simulink model "Impedance_Gantry_Model_V3"  (R2021b)
settings: Solver=VariableStepAuto  StartTime=0  StopTime=5  FixedStep=0.001  RelTol=1e-3  AbsTol=1e-3  EnableMultiTasking=on
values from neighbouring files (symbols this model uses):
  Fmin = obj_x*obj_y*obj_z*obj_density*9.81/obj_coeff/obj_contactpt    (= 4.90500000153)    [Impedance_Control_V1.m]    (also in Impedance_Control_V2.m; Impedance_Control_V3.m; Impedance_Control_V4.m; Impedance_Control_V5.m)
  N = 100    [Gantry_Model_Sim_V1.m]    (also in Impedance_Control_V1.m = 10; Impedance_Control_V2.m = 10; Impedance_Control_V3.m = 40; Impedance_Control_V3_plot.m = 40)
  Ts = 0.01    [Gantry_Model_Sim_V1.m]    (also in Impedance_Control_V1.m = 0.0125; Impedance_Control_V2.m = 0.0125; Impedance_Control_V3.m = 0.0125; Impedance_Control_V4.m = 0.0125)
  z_clear = 1    [Impedance_Control_V1.m]    (also in Impedance_Control_V2.m; Impedance_Control_V3.m; Impedance_Control_V4.m; Impedance_Control_V5.m)
undefined symbols (not defined in the file or in its folder): X, Y, Z
libraries: sm_lib x89, nesl_utility x14, slpidlib x7
(part 3 of 4)

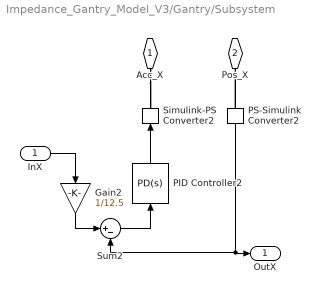
== system Impedance_Gantry_Model_V3/Gantry/Subsystem ==
  InX : Inport
  Gain2 : Gain  Gain=1/12.5
  PID Controller2 : slpidlib/PID Controller  Controller=PD  Form=Parallel  TimeDomain=Continuous-time  UseExternalTs=off  SampleTime=-1  IntegratorMethod=Forward Euler  FilterMethod=Forward Euler  ControllerParametersSource=internal  P=27146.6747627399  I=4557008.73655903  D=1020.02839756073  UseFilter=on  N=1838.86945148368  TunerSelectOption=Transfer Function Based (PID Tuner App)  InitialConditionSource=internal  InitialConditionForIntegrator=0  InitialConditionForFilter=0  DifferentiatorICPrevScaledInput=0  ExternalReset=none  TrackingMode=off  Kt=1  LimitOutput=off  SatLimitsSource=internal  UpperSaturationLimit=inf  LowerSaturationLimit=-inf  LinearizeAsGain=on  AntiWindupMode=none  Kb=1  POutMin=[]  POutMax=[]  IOutMin=[]  IOutMax=[]  DOutMin=[]  DOutMax=[]  NOutMin=[]  NOutMax=[]  SumOutMin=[]  SumOutMax=[]  SaturationOutMin=[]  SaturationOutMax=[]  PParamMin=[]  PParamMax=[]  IParamMin=[]  IParamMax=[]  DParamMin=[]  DParamMax=[]  NParamMin=[]  NParamMax=[]  KbParamMin=[]  KbParamMax=[]  KtParamMin=[]  KtParamMax=[]  KbOutMin=[]  KbOutMax=[]  KtOutMin=[]  KtOutMax=[]  IntegratorOutMin=[]  IntegratorOutMax=[]  FilterOutMin=[]  FilterOutMax=[]  SumI1OutMin=[]  SumI1OutMax=[]  SumI2OutMin=[]  SumI2OutMax=[]  SumI3OutMin=[]  SumI3OutMax=[]  SumI4OutMin=[]  SumI4OutMax=[]  SumDOutMin=[]  SumDOutMax=[]  DifferentiatorOutMin=[]  DifferentiatorOutMax=[]  FilterDiffOutCoefMin=[]  FilterDiffOutCoefMax=[]  ReciprocalOutMin=[]  ReciprocalOutMax=[]  SumDenOutMin=[]  SumDenOutMax=[]  SumNumOutMin=[]  SumNumOutMax=[]  DivideOutMin=[]  DivideOutMax=[]  UdiffTsProdOutMin=[]  UdiffTsProdOutMax=[]  NTsProdOutMin=[]  NTsProdOutMax=[]  UintegralTsProdOutMin=[]  UintegralTsProdOutMax=[]  UngainTsProdOutMin=[]  UngainTsProdOutMax=[]  IntegratorContinuousStateAttributes=''  IntegratorStateMustResolveToSignalObject=off  IntegratorRTWStateStorageClass=Auto  FilterContinuousStateAttributes=''  FilterStateMustResolveToSignalObject=off  FilterRTWStateStorageClass=Auto  ParallelPVariant=InternalParameters  IdealPVariant=Disabled  IVariant=Disabled  DVariant=InternalParameters  IntegratorVariant=Disabled  SatVariant=Disabled  AWVariant=Disabled  PCopyVariant=Disabled  TRVariant=Disabled  FdbkBlocksVariant=Forward  IdealPFdbkVariant=Disabled  SatFdbkVariant=Disabled  DerivativeFilterVariant=ContFilter  NVariant=InternalParameters  NCopyVariant=Disabled  FilterICVariant=InternalICsFilter  IntegratorICVariant=Disabled  ExternalResetVariant=Disabled  TRSumVariant=Passthrough  SumFdbkVariant=Disabled  SumVariant=Sum_PD  TsampFilterVariant=InternalTs  TsampNgainVariant=Passthrough  TsampIntegralVariant=Disabled_SignalSpec  ExternalSaturationOutDataTypeStr=Inherit: Same as second input
  PS-Simulink Converter2 : nesl_utility/PS-Simulink Converter  PhysicalDomain=network_engine_domain  SubClassName=ps_output  LeftPortType=input  RightPortType=output  PseudoPeriodic=off  Frequencies=[]  Unit=inherit  AffineConversion=off
      settings: SourceProductBaseCode=PW,SS
  Simulink-PS Converter2 : nesl_utility/Simulink-PS Converter  PhysicalDomain=network_engine_domain  SubClassName=ps_input  LeftPortType=input  RightPortType=output  PseudoPeriodic=off  Frequencies=[]  NoiseDistribution=none  NoiseParameters=[]  Unit=1  AffineConversion=off  FilteringAndDerivatives=provide  SimscapeFilterOrder=1  InputFilterTimeConstant=0.001  UdotUserProvided=0
      settings: SourceProductBaseCode=PW,SS
  Sum2 : Sum  Inputs=|+-
  Acc_X : PMIOPort  Side=Left
  Pos_X : PMIOPort  Port=2  Side=Right
  OutX : Outport
  wires:
  InX/1 -> Gain2/1
  PS-Simulink Converter2/1 -> OutX/1, Sum2/2
  Sum2/1 -> PID Controller2/1
  PID Controller2/1 -> Simulink-PS Converter2/1
  Gain2/1 -> Sum2/1
  connections:
  PS-Simulink Converter2/LConn1 -- Pos_X/RConn1
  Acc_X/RConn1 -- Simulink-PS Converter2/RConn1

== system Impedance_Gantry_Model_V3/Gantry/Y axis dynamics ==
  InY : Inport
  Gain1 : Gain  Gain=1/500
  PID Controller1 : slpidlib/PID Controller  Controller=PD  Form=Parallel  TimeDomain=Continuous-time  UseExternalTs=off  SampleTime=-1  IntegratorMethod=Forward Euler  FilterMethod=Forward Euler  ControllerParametersSource=internal  P=131139.225952649  I=4557008.73655903  D=1480.57986826149  UseFilter=on  N=47126.9268470762  TunerSelectOption=Transfer Function Based (PID Tuner App)  InitialConditionSource=internal  InitialConditionForIntegrator=0  InitialConditionForFilter=0  DifferentiatorICPrevScaledInput=0  ExternalReset=none  TrackingMode=off  Kt=1  LimitOutput=off  SatLimitsSource=internal  UpperSaturationLimit=inf  LowerSaturationLimit=-inf  LinearizeAsGain=on  AntiWindupMode=none  Kb=1  POutMin=[]  POutMax=[]  IOutMin=[]  IOutMax=[]  DOutMin=[]  DOutMax=[]  NOutMin=[]  NOutMax=[]  SumOutMin=[]  SumOutMax=[]  SaturationOutMin=[]  SaturationOutMax=[]  PParamMin=[]  PParamMax=[]  IParamMin=[]  IParamMax=[]  DParamMin=[]  DParamMax=[]  NParamMin=[]  NParamMax=[]  KbParamMin=[]  KbParamMax=[]  KtParamMin=[]  KtParamMax=[]  KbOutMin=[]  KbOutMax=[]  KtOutMin=[]  KtOutMax=[]  IntegratorOutMin=[]  IntegratorOutMax=[]  FilterOutMin=[]  FilterOutMax=[]  SumI1OutMin=[]  SumI1OutMax=[]  SumI2OutMin=[]  SumI2OutMax=[]  SumI3OutMin=[]  SumI3OutMax=[]  SumI4OutMin=[]  SumI4OutMax=[]  SumDOutMin=[]  SumDOutMax=[]  DifferentiatorOutMin=[]  DifferentiatorOutMax=[]  FilterDiffOutCoefMin=[]  FilterDiffOutCoefMax=[]  ReciprocalOutMin=[]  ReciprocalOutMax=[]  SumDenOutMin=[]  SumDenOutMax=[]  SumNumOutMin=[]  SumNumOutMax=[]  DivideOutMin=[]  DivideOutMax=[]  UdiffTsProdOutMin=[]  UdiffTsProdOutMax=[]  NTsProdOutMin=[]  NTsProdOutMax=[]  UintegralTsProdOutMin=[]  UintegralTsProdOutMax=[]  UngainTsProdOutMin=[]  UngainTsProdOutMax=[]  IntegratorContinuousStateAttributes=''  IntegratorStateMustResolveToSignalObject=off  IntegratorRTWStateStorageClass=Auto  FilterContinuousStateAttributes=''  FilterStateMustResolveToSignalObject=off  FilterRTWStateStorageClass=Auto  ParallelPVariant=InternalParameters  IdealPVariant=Disabled  IVariant=Disabled  DVariant=InternalParameters  IntegratorVariant=Disabled  SatVariant=Disabled  AWVariant=Disabled  PCopyVariant=Disabled  TRVariant=Disabled  FdbkBlocksVariant=Forward  IdealPFdbkVariant=Disabled  SatFdbkVariant=Disabled  DerivativeFilterVariant=ContFilter  NVariant=InternalParameters  NCopyVariant=Disabled  FilterICVariant=InternalICsFilter  IntegratorICVariant=Disabled  ExternalResetVariant=Disabled  TRSumVariant=Passthrough  SumFdbkVariant=Disabled  SumVariant=Sum_PD  TsampFilterVariant=InternalTs  TsampNgainVariant=Passthrough  TsampIntegralVariant=Disabled_SignalSpec  ExternalSaturationOutDataTypeStr=Inherit: Same as second input
  PS-Simulink Converter1 : nesl_utility/PS-Simulink Converter  PhysicalDomain=network_engine_domain  SubClassName=ps_output  LeftPortType=input  RightPortType=output  PseudoPeriodic=off  Frequencies=[]  Unit=inherit  AffineConversion=off
      settings: SourceProductBaseCode=PW,SS
  Simulink-PS Converter1 : nesl_utility/Simulink-PS Converter  PhysicalDomain=network_engine_domain  SubClassName=ps_input  LeftPortType=input  RightPortType=output  PseudoPeriodic=off  Frequencies=[]  NoiseDistribution=none  NoiseParameters=[]  Unit=1  AffineConversion=off  FilteringAndDerivatives=provide  SimscapeFilterOrder=1  InputFilterTimeConstant=0.001  UdotUserProvided=0
      settings: SourceProductBaseCode=PW,SS
  Sum1 : Sum  Inputs=|+-
  Acc_Y : PMIOPort  Side=Left
  Pos_Y : PMIOPort  Port=2  Side=Right
  OutY : Outport
  wires:
  Gain1/1 -> Sum1/1
  PID Controller1/1 -> Simulink-PS Converter1/1
  PS-Simulink Converter1/1 -> Sum1/2, OutY/1
  InY/1 -> Gain1/1
  Sum1/1 -> PID Controller1/1
  connections:
  Pos_Y/RConn1 -- PS-Simulink Converter1/LConn1
  Simulink-PS Converter1/RConn1 -- Acc_Y/RConn1

== system Impedance_Gantry_Model_V3/Gantry/Z axis dynamics ==
  InZ : Inport
  Gain : Gain  Gain=1/1550.672269
  PID Controller : slpidlib/PID Controller  Controller=PD  Form=Parallel  TimeDomain=Continuous-time  UseExternalTs=off  SampleTime=-1  IntegratorMethod=Forward Euler  FilterMethod=Forward Euler  ControllerParametersSource=internal  P=33734.3806  I=809967.572319892  D=163.3421  UseFilter=on  N=13723.0524  TunerSelectOption=Transfer Function Based (PID Tuner App)  InitialConditionSource=internal  InitialConditionForIntegrator=0  InitialConditionForFilter=0  DifferentiatorICPrevScaledInput=0  ExternalReset=none  TrackingMode=off  Kt=1  LimitOutput=off  SatLimitsSource=internal  UpperSaturationLimit=inf  LowerSaturationLimit=-inf  LinearizeAsGain=on  AntiWindupMode=none  Kb=1  POutMin=[]  POutMax=[]  IOutMin=[]  IOutMax=[]  DOutMin=[]  DOutMax=[]  NOutMin=[]  NOutMax=[]  SumOutMin=[]  SumOutMax=[]  SaturationOutMin=[]  SaturationOutMax=[]  PParamMin=[]  PParamMax=[]  IParamMin=[]  IParamMax=[]  DParamMin=[]  DParamMax=[]  NParamMin=[]  NParamMax=[]  KbParamMin=[]  KbParamMax=[]  KtParamMin=[]  KtParamMax=[]  KbOutMin=[]  KbOutMax=[]  KtOutMin=[]  KtOutMax=[]  IntegratorOutMin=[]  IntegratorOutMax=[]  FilterOutMin=[]  FilterOutMax=[]  SumI1OutMin=[]  SumI1OutMax=[]  SumI2OutMin=[]  SumI2OutMax=[]  SumI3OutMin=[]  SumI3OutMax=[]  SumI4OutMin=[]  SumI4OutMax=[]  SumDOutMin=[]  SumDOutMax=[]  DifferentiatorOutMin=[]  DifferentiatorOutMax=[]  FilterDiffOutCoefMin=[]  FilterDiffOutCoefMax=[]  ReciprocalOutMin=[]  ReciprocalOutMax=[]  SumDenOutMin=[]  SumDenOutMax=[]  SumNumOutMin=[]  SumNumOutMax=[]  DivideOutMin=[]  DivideOutMax=[]  UdiffTsProdOutMin=[]  UdiffTsProdOutMax=[]  NTsProdOutMin=[]  NTsProdOutMax=[]  UintegralTsProdOutMin=[]  UintegralTsProdOutMax=[]  UngainTsProdOutMin=[]  UngainTsProdOutMax=[]  IntegratorContinuousStateAttributes=''  IntegratorStateMustResolveToSignalObject=off  IntegratorRTWStateStorageClass=Auto  FilterContinuousStateAttributes=''  FilterStateMustResolveToSignalObject=off  FilterRTWStateStorageClass=Auto  ParallelPVariant=InternalParameters  IdealPVariant=Disabled  IVariant=Disabled  DVariant=InternalParameters  IntegratorVariant=Disabled  SatVariant=Disabled  AWVariant=Disabled  PCopyVariant=Disabled  TRVariant=Disabled  FdbkBlocksVariant=Forward  IdealPFdbkVariant=Disabled  SatFdbkVariant=Disabled  DerivativeFilterVariant=ContFilter  NVariant=InternalParameters  NCopyVariant=Disabled  FilterICVariant=InternalICsFilter  IntegratorICVariant=Disabled  ExternalResetVariant=Disabled  TRSumVariant=Passthrough  SumFdbkVariant=Disabled  SumVariant=Sum_PD  TsampFilterVariant=InternalTs  TsampNgainVariant=Passthrough  TsampIntegralVariant=Disabled_SignalSpec  ExternalSaturationOutDataTypeStr=Inherit: Same as second input
  PS-Simulink Converter : nesl_utility/PS-Simulink Converter  PhysicalDomain=network_engine_domain  SubClassName=ps_output  LeftPortType=input  RightPortType=output  PseudoPeriodic=off  Frequencies=[]  Unit=inherit  AffineConversion=off
      settings: SourceProductBaseCode=PW,SS
  Simulink-PS Converter : nesl_utility/Simulink-PS Converter  PhysicalDomain=network_engine_domain  SubClassName=ps_input  LeftPortType=input  RightPortType=output  PseudoPeriodic=off  Frequencies=[]  NoiseDistribution=none  NoiseParameters=[]  Unit=1  AffineConversion=off  FilteringAndDerivatives=provide  SimscapeFilterOrder=1  InputFilterTimeConstant=0.001  UdotUserProvided=0
      settings: SourceProductBaseCode=PW,SS
  Sum : Sum  Inputs=|+-
  Acc_Z : PMIOPort  Side=Left
  Pos_Z : PMIOPort  Port=2  Side=Right
  OutZ : Outport
  wires:
  Sum/1 -> PID Controller/1
  PS-Simulink Converter/1 -> OutZ/1, Sum/2
  PID Controller/1 -> Simulink-PS Converter/1
  Gain/1 -> Sum/1
  InZ/1 -> Gain/1
  connections:
  PS-Simulink Converter/LConn1 -- Pos_Z/RConn1
  Simulink-PS Converter/RConn1 -- Acc_Z/RConn1

== system Impedance_Gantry_Model_V3/Gantry/Z axis dynamics1 ==
  InZ : Inport
  Gain : Gain  Gain=1/1550.672269
  PID Controller : slpidlib/PID Controller  Controller=PD  Form=Parallel  TimeDomain=Continuous-time  UseExternalTs=off  SampleTime=-1  IntegratorMethod=Forward Euler  FilterMethod=Forward Euler  ControllerParametersSource=internal  P=33734.3806  I=809967.572319892  D=163.3421  UseFilter=on  N=13723.0524  TunerSelectOption=Transfer Function Based (PID Tuner App)  InitialConditionSource=internal  InitialConditionForIntegrator=0  InitialConditionForFilter=0  DifferentiatorICPrevScaledInput=0  ExternalReset=none  TrackingMode=off  Kt=1  LimitOutput=off  SatLimitsSource=internal  UpperSaturationLimit=inf  LowerSaturationLimit=-inf  LinearizeAsGain=on  AntiWindupMode=none  Kb=1  POutMin=[]  POutMax=[]  IOutMin=[]  IOutMax=[]  DOutMin=[]  DOutMax=[]  NOutMin=[]  NOutMax=[]  SumOutMin=[]  SumOutMax=[]  SaturationOutMin=[]  SaturationOutMax=[]  PParamMin=[]  PParamMax=[]  IParamMin=[]  IParamMax=[]  DParamMin=[]  DParamMax=[]  NParamMin=[]  NParamMax=[]  KbParamMin=[]  KbParamMax=[]  KtParamMin=[]  KtParamMax=[]  KbOutMin=[]  KbOutMax=[]  KtOutMin=[]  KtOutMax=[]  IntegratorOutMin=[]  IntegratorOutMax=[]  FilterOutMin=[]  FilterOutMax=[]  SumI1OutMin=[]  SumI1OutMax=[]  SumI2OutMin=[]  SumI2OutMax=[]  SumI3OutMin=[]  SumI3OutMax=[]  SumI4OutMin=[]  SumI4OutMax=[]  SumDOutMin=[]  SumDOutMax=[]  DifferentiatorOutMin=[]  DifferentiatorOutMax=[]  FilterDiffOutCoefMin=[]  FilterDiffOutCoefMax=[]  ReciprocalOutMin=[]  ReciprocalOutMax=[]  SumDenOutMin=[]  SumDenOutMax=[]  SumNumOutMin=[]  SumNumOutMax=[]  DivideOutMin=[]  DivideOutMax=[]  UdiffTsProdOutMin=[]  UdiffTsProdOutMax=[]  NTsProdOutMin=[]  NTsProdOutMax=[]  UintegralTsProdOutMin=[]  UintegralTsProdOutMax=[]  UngainTsProdOutMin=[]  UngainTsProdOutMax=[]  IntegratorContinuousStateAttributes=''  IntegratorStateMustResolveToSignalObject=off  IntegratorRTWStateStorageClass=Auto  FilterContinuousStateAttributes=''  FilterStateMustResolveToSignalObject=off  FilterRTWStateStorageClass=Auto  ParallelPVariant=InternalParameters  IdealPVariant=Disabled  IVariant=Disabled  DVariant=InternalParameters  IntegratorVariant=Disabled  SatVariant=Disabled  AWVariant=Disabled  PCopyVariant=Disabled  TRVariant=Disabled  FdbkBlocksVariant=Forward  IdealPFdbkVariant=Disabled  SatFdbkVariant=Disabled  DerivativeFilterVariant=ContFilter  NVariant=InternalParameters  NCopyVariant=Disabled  FilterICVariant=InternalICsFilter  IntegratorICVariant=Disabled  ExternalResetVariant=Disabled  TRSumVariant=Passthrough  SumFdbkVariant=Disabled  SumVariant=Sum_PD  TsampFilterVariant=InternalTs  TsampNgainVariant=Passthrough  TsampIntegralVariant=Disabled_SignalSpec  ExternalSaturationOutDataTypeStr=Inherit: Same as second input
  PS-Simulink Converter : nesl_utility/PS-Simulink Converter  PhysicalDomain=network_engine_domain  SubClassName=ps_output  LeftPortType=input  RightPortType=output  PseudoPeriodic=off  Frequencies=[]  Unit=inherit  AffineConversion=off
      settings: SourceProductBaseCode=PW,SS
  Simulink-PS Converter : nesl_utility/Simulink-PS Converter  PhysicalDomain=network_engine_domain  SubClassName=ps_input  LeftPortType=input  RightPortType=output  PseudoPeriodic=off  Frequencies=[]  NoiseDistribution=none  NoiseParameters=[]  Unit=1  AffineConversion=off  FilteringAndDerivatives=provide  SimscapeFilterOrder=1  InputFilterTimeConstant=0.001  UdotUserProvided=0
      settings: SourceProductBaseCode=PW,SS
  Sum : Sum  Inputs=|+-
  Acc_Z : PMIOPort  Side=Left
  Pos_Z : PMIOPort  Port=2  Side=Right
  OutZ : Outport
  wires:
  Sum/1 -> PID Controller/1
  PS-Simulink Converter/1 -> OutZ/1, Sum/2
  PID Controller/1 -> Simulink-PS Converter/1
  Gain/1 -> Sum/1
  InZ/1 -> Gain/1
  connections:
  PS-Simulink Converter/LConn1 -- Pos_Z/RConn1
  Simulink-PS Converter/RConn1 -- Acc_Z/RConn1

== system Impedance_Gantry_Model_V3/Gantry/Z axis dynamics2 ==
  InZ : Inport
  Gain : Gain  Gain=1/1550.672269
  PID Controller : slpidlib/PID Controller  Controller=PD  Form=Parallel  TimeDomain=Continuous-time  UseExternalTs=off  SampleTime=-1  IntegratorMethod=Forward Euler  FilterMethod=Forward Euler  ControllerParametersSource=internal  P=33734.3806  I=809967.572319892  D=163.3421  UseFilter=on  N=13723.0524  TunerSelectOption=Transfer Function Based (PID Tuner App)  InitialConditionSource=internal  InitialConditionForIntegrator=0  InitialConditionForFilter=0  DifferentiatorICPrevScaledInput=0  ExternalReset=none  TrackingMode=off  Kt=1  LimitOutput=off  SatLimitsSource=internal  UpperSaturationLimit=inf  LowerSaturationLimit=-inf  LinearizeAsGain=on  AntiWindupMode=none  Kb=1  POutMin=[]  POutMax=[]  IOutMin=[]  IOutMax=[]  DOutMin=[]  DOutMax=[]  NOutMin=[]  NOutMax=[]  SumOutMin=[]  SumOutMax=[]  SaturationOutMin=[]  SaturationOutMax=[]  PParamMin=[]  PParamMax=[]  IParamMin=[]  IParamMax=[]  DParamMin=[]  DParamMax=[]  NParamMin=[]  NParamMax=[]  KbParamMin=[]  KbParamMax=[]  KtParamMin=[]  KtParamMax=[]  KbOutMin=[]  KbOutMax=[]  KtOutMin=[]  KtOutMax=[]  IntegratorOutMin=[]  IntegratorOutMax=[]  FilterOutMin=[]  FilterOutMax=[]  SumI1OutMin=[]  SumI1OutMax=[]  SumI2OutMin=[]  SumI2OutMax=[]  SumI3OutMin=[]  SumI3OutMax=[]  SumI4OutMin=[]  SumI4OutMax=[]  SumDOutMin=[]  SumDOutMax=[]  DifferentiatorOutMin=[]  DifferentiatorOutMax=[]  FilterDiffOutCoefMin=[]  FilterDiffOutCoefMax=[]  ReciprocalOutMin=[]  ReciprocalOutMax=[]  SumDenOutMin=[]  SumDenOutMax=[]  SumNumOutMin=[]  SumNumOutMax=[]  DivideOutMin=[]  DivideOutMax=[]  UdiffTsProdOutMin=[]  UdiffTsProdOutMax=[]  NTsProdOutMin=[]  NTsProdOutMax=[]  UintegralTsProdOutMin=[]  UintegralTsProdOutMax=[]  UngainTsProdOutMin=[]  UngainTsProdOutMax=[]  IntegratorContinuousStateAttributes=''  IntegratorStateMustResolveToSignalObject=off  IntegratorRTWStateStorageClass=Auto  FilterContinuousStateAttributes=''  FilterStateMustResolveToSignalObject=off  FilterRTWStateStorageClass=Auto  ParallelPVariant=InternalParameters  IdealPVariant=Disabled  IVariant=Disabled  DVariant=InternalParameters  IntegratorVariant=Disabled  SatVariant=Disabled  AWVariant=Disabled  PCopyVariant=Disabled  TRVariant=Disabled  FdbkBlocksVariant=Forward  IdealPFdbkVariant=Disabled  SatFdbkVariant=Disabled  DerivativeFilterVariant=ContFilter  NVariant=InternalParameters  NCopyVariant=Disabled  FilterICVariant=InternalICsFilter  IntegratorICVariant=Disabled  ExternalResetVariant=Disabled  TRSumVariant=Passthrough  SumFdbkVariant=Disabled  SumVariant=Sum_PD  TsampFilterVariant=InternalTs  TsampNgainVariant=Passthrough  TsampIntegralVariant=Disabled_SignalSpec  ExternalSaturationOutDataTypeStr=Inherit: Same as second input
  PS-Simulink Converter : nesl_utility/PS-Simulink Converter  PhysicalDomain=network_engine_domain  SubClassName=ps_output  LeftPortType=input  RightPortType=output  PseudoPeriodic=off  Frequencies=[]  Unit=inherit  AffineConversion=off
      settings: SourceProductBaseCode=PW,SS
  Simulink-PS Converter : nesl_utility/Simulink-PS Converter  PhysicalDomain=network_engine_domain  SubClassName=ps_input  LeftPortType=input  RightPortType=output  PseudoPeriodic=off  Frequencies=[]  NoiseDistribution=none  NoiseParameters=[]  Unit=1  AffineConversion=off  FilteringAndDerivatives=provide  SimscapeFilterOrder=1  InputFilterTimeConstant=0.001  UdotUserProvided=0
      settings: SourceProductBaseCode=PW,SS
  Sum : Sum  Inputs=|+-
  Acc_Z : PMIOPort  Side=Left
  Pos_Z : PMIOPort  Port=2  Side=Right
  OutZ : Outport
  wires:
  Sum/1 -> PID Controller/1
  PS-Simulink Converter/1 -> OutZ/1, Sum/2
  PID Controller/1 -> Simulink-PS Converter/1
  Gain/1 -> Sum/1
  InZ/1 -> Gain/1
  connections:
  PS-Simulink Converter/LConn1 -- Pos_Z/RConn1
  Simulink-PS Converter/RConn1 -- Acc_Z/RConn1

== system Impedance_Gantry_Model_V3/ObjectAndEnviroment/BBL ==
  BBL : sm_lib/Frames and Transforms/Rigid Transform  TranslationMethod=Cartesian  TranslationStandardOffset=0  TranslationLengthUnit=mm  TranslationStandardAxis=+Z  TranslationCartesianOffset=[25 25 0]  TranslationROffset=0  TranslationROffsetUnits=m  TranslationZOffset=0  TranslationZOffsetUnits=m  TranslationThetaOffset=0  TranslationThetaOffsetUnits=deg  RotationMethod=None  RotationAngleUnits=deg  RotationStandardAxis=+Z  RotationAngle=0.0  RotationArbitraryAxis=[0 0 1]  FollAlignAxisA=+X  BaseAlignAxisA=+Y  FollAlignAxisB=+Y  BaseAlignAxisB=+Z  RotationSequenceAxes=FollowerAxes  RotationSequence=XYX  RotationSequenceAngles=[0 0 0]  RotationSequenceAnglesUnits=deg  RotationMatrix=[1 0 0; 0 1 0; 0 0 1]
  BBLBall : sm_lib/Body Elements/Spherical Solid  GraphicAmbientColor=[0.15 0.15 0.15 1.0]  BasedOnType=Density  CenterOfMass=[0 0 0]  CenterOfMassUnits=m  GraphicDiffuseColor=[0.5 0.5 0.5]  Density=1000  DensityUnits=kg/m^3  DoExposeReferenceFrame=on  GraphicEmissiveColor=[0.0 0.0 0.0 1.0]  ExportEntireGeometry=on  SerializedExposedGeometries=<ExposedGeometries><ExposedGeometry><RawGeometryId>entire</RawGeometryId><ExposedGeometryId>G</ExposedGeometryId></ExposedGeometry></ExposedGeometries>  SerializedFrames=<Frames/>  MarkerShape=Sphere  MarkerSize=10  GraphicType=FromGeometry  InertiaType=CalculateFromGeometry  Mass=1  MassUnits=kg  MomentsOfInertia=[1 1 1]  MomentsOfInertiaUnits=kg*m^2  GraphicOpacity=1.0  ProductsOfInertia=[0 0 0]  ProductsOfInertiaUnits=kg*m^2  GraphicShininess=75  GraphicSpecularColor=[0.5 0.5 0.5 1.0]  SphereRadius=1  SphereRadiusUnits=mm  GraphicVisPropType=SimpleVisualProperties
  BBLConveyerDest : sm_lib/Forces and Torques/Spatial Contact Force  CoefficientOfDynamicFriction=0.5  CoefficientOfStaticFriction=0.5  SenseContactBaseRotation=off  SenseContactBaseTranslation=off  NormalDamping=30  NormalDampingUnits=N/(m/s)  SenseContactFollowerRotation=off  SenseContactFollowerTranslation=off  SenseContactSignal=off  NormalStiffness=1e4  NormalStiffnessUnits=N/m  FrictionalCriticalVelocity=1e-3  FrictionalCriticalVelocityUnits=m/s  ZeroCrossDetectContactStartAndEnd=off  FrictionType=SmoothStickSlip  SenseFrictionalForceMagnitude=off  SenseNormalForceMagnitude=off  NormalForceType=SmoothSpringDamper  SenseNormalVelocity=off  SenseSeparationDistance=off  SenseTangentialVelocity=off  SenseTangentialVelocityMagnitude=off  NormalTransitionRegionWidth=1e-5  NormalTransitionRegionWidthUnits=m
  BBLConveyerOri : sm_lib/Forces and Torques/Spatial Contact Force  CoefficientOfDynamicFriction=0.5  CoefficientOfStaticFriction=0.5  SenseContactBaseRotation=off  SenseContactBaseTranslation=off  NormalDamping=30  NormalDampingUnits=N/(m/s)  SenseContactFollowerRotation=off  SenseContactFollowerTranslation=off  SenseContactSignal=off  NormalStiffness=1e4  NormalStiffnessUnits=N/m  FrictionalCriticalVelocity=1e-3  FrictionalCriticalVelocityUnits=m/s  ZeroCrossDetectContactStartAndEnd=off  FrictionType=SmoothStickSlip  SenseFrictionalForceMagnitude=off  SenseNormalForceMagnitude=off  NormalForceType=SmoothSpringDamper  SenseNormalVelocity=off  SenseSeparationDistance=off  SenseTangentialVelocity=off  SenseTangentialVelocityMagnitude=off  NormalTransitionRegionWidth=1e-5  NormalTransitionRegionWidthUnits=m
  BBLGripper : sm_lib/Forces and Torques/Spatial Contact Force  CoefficientOfDynamicFriction=0.5  CoefficientOfStaticFriction=0.5  SenseContactBaseRotation=off  SenseContactBaseTranslation=off  NormalDamping=0  NormalDampingUnits=N/(m/s)  SenseContactFollowerRotation=off  SenseContactFollowerTranslation=off  SenseContactSignal=off  NormalStiffness=1e4  NormalStiffnessUnits=N/m  FrictionalCriticalVelocity=1e-3  FrictionalCriticalVelocityUnits=m/s  ZeroCrossDetectContactStartAndEnd=off  FrictionType=SmoothStickSlip  SenseFrictionalForceMagnitude=off  SenseNormalForceMagnitude=off  NormalForceType=SmoothSpringDamper  SenseNormalVelocity=off  SenseSeparationDistance=off  SenseTangentialVelocity=off  SenseTangentialVelocityMagnitude=off  NormalTransitionRegionWidth=1e-5  NormalTransitionRegionWidthUnits=m
  Obj : PMIOPort  Side=Left
  Gripper : PMIOPort  Port=2  Side=Right
  ConveyerOri : PMIOPort  Port=3  Side=Right
  ConveyerDest : PMIOPort  Port=4  Side=Right
  connections:
  BBLBall/LConn1 -- BBLConveyerDest/LConn1 -- BBLConveyerOri/LConn1 -- BBLGripper/LConn1
  BBL/LConn1 -- Obj/RConn1
  BBLBall/RConn1 -- BBL/RConn1
  ConveyerOri/RConn1 -- BBLConveyerOri/RConn1
  BBLGripper/RConn1 -- Gripper/RConn1
  BBLConveyerDest/RConn1 -- ConveyerDest/RConn1

== system Impedance_Gantry_Model_V3/ObjectAndEnviroment/BRR ==
  BBR : sm_lib/Frames and Transforms/Rigid Transform  TranslationMethod=Cartesian  TranslationStandardOffset=0  TranslationLengthUnit=mm  TranslationStandardAxis=+Z  TranslationCartesianOffset=[25 0 0]  TranslationROffset=0  TranslationROffsetUnits=m  TranslationZOffset=0  TranslationZOffsetUnits=m  TranslationThetaOffset=0  TranslationThetaOffsetUnits=deg  RotationMethod=None  RotationAngleUnits=deg  RotationStandardAxis=+Z  RotationAngle=0.0  RotationArbitraryAxis=[0 0 1]  FollAlignAxisA=+X  BaseAlignAxisA=+Y  FollAlignAxisB=+Y  BaseAlignAxisB=+Z  RotationSequenceAxes=FollowerAxes  RotationSequence=XYX  RotationSequenceAngles=[0 0 0]  RotationSequenceAnglesUnits=deg  RotationMatrix=[1 0 0; 0 1 0; 0 0 1]
  BBRBall : sm_lib/Body Elements/Spherical Solid  GraphicAmbientColor=[0.15 0.15 0.15 1.0]  BasedOnType=Density  CenterOfMass=[0 0 0]  CenterOfMassUnits=m  GraphicDiffuseColor=[0.5 0.5 0.5]  Density=1000  DensityUnits=kg/m^3  DoExposeReferenceFrame=on  GraphicEmissiveColor=[0.0 0.0 0.0 1.0]  ExportEntireGeometry=on  SerializedExposedGeometries=<ExposedGeometries><ExposedGeometry><RawGeometryId>entire</RawGeometryId><ExposedGeometryId>G</ExposedGeometryId></ExposedGeometry></ExposedGeometries>  SerializedFrames=<Frames/>  MarkerShape=Sphere  MarkerSize=10  GraphicType=FromGeometry  InertiaType=CalculateFromGeometry  Mass=1  MassUnits=kg  MomentsOfInertia=[1 1 1]  MomentsOfInertiaUnits=kg*m^2  GraphicOpacity=1.0  ProductsOfInertia=[0 0 0]  ProductsOfInertiaUnits=kg*m^2  GraphicShininess=75  GraphicSpecularColor=[0.5 0.5 0.5 1.0]  SphereRadius=1  SphereRadiusUnits=mm  GraphicVisPropType=SimpleVisualProperties
  BBRConveyerDest : sm_lib/Forces and Torques/Spatial Contact Force  CoefficientOfDynamicFriction=0.5  CoefficientOfStaticFriction=0.5  SenseContactBaseRotation=off  SenseContactBaseTranslation=off  NormalDamping=30  NormalDampingUnits=N/(m/s)  SenseContactFollowerRotation=off  SenseContactFollowerTranslation=off  SenseContactSignal=off  NormalStiffness=1e4  NormalStiffnessUnits=N/m  FrictionalCriticalVelocity=1e-3  FrictionalCriticalVelocityUnits=m/s  ZeroCrossDetectContactStartAndEnd=off  FrictionType=SmoothStickSlip  SenseFrictionalForceMagnitude=off  SenseNormalForceMagnitude=off  NormalForceType=SmoothSpringDamper  SenseNormalVelocity=off  SenseSeparationDistance=off  SenseTangentialVelocity=off  SenseTangentialVelocityMagnitude=off  NormalTransitionRegionWidth=1e-5  NormalTransitionRegionWidthUnits=m
  BBRConveyerOri : sm_lib/Forces and Torques/Spatial Contact Force  CoefficientOfDynamicFriction=0.5  CoefficientOfStaticFriction=0.5  SenseContactBaseRotation=off  SenseContactBaseTranslation=off  NormalDamping=30  NormalDampingUnits=N/(m/s)  SenseContactFollowerRotation=off  SenseContactFollowerTranslation=off  SenseContactSignal=off  NormalStiffness=1e4  NormalStiffnessUnits=N/m  FrictionalCriticalVelocity=1e-3  FrictionalCriticalVelocityUnits=m/s  ZeroCrossDetectContactStartAndEnd=off  FrictionType=SmoothStickSlip  SenseFrictionalForceMagnitude=off  SenseNormalForceMagnitude=off  NormalForceType=SmoothSpringDamper  SenseNormalVelocity=off  SenseSeparationDistance=off  SenseTangentialVelocity=off  SenseTangentialVelocityMagnitude=off  NormalTransitionRegionWidth=1e-5  NormalTransitionRegionWidthUnits=m
  BBRGripper : sm_lib/Forces and Torques/Spatial Contact Force  CoefficientOfDynamicFriction=0.5  CoefficientOfStaticFriction=0.5  SenseContactBaseRotation=off  SenseContactBaseTranslation=off  NormalDamping=0  NormalDampingUnits=N/(m/s)  SenseContactFollowerRotation=off  SenseContactFollowerTranslation=off  SenseContactSignal=off  NormalStiffness=1e4  NormalStiffnessUnits=N/m  FrictionalCriticalVelocity=1e-3  FrictionalCriticalVelocityUnits=m/s  ZeroCrossDetectContactStartAndEnd=off  FrictionType=SmoothStickSlip  SenseFrictionalForceMagnitude=off  SenseNormalForceMagnitude=off  NormalForceType=SmoothSpringDamper  SenseNormalVelocity=off  SenseSeparationDistance=off  SenseTangentialVelocity=off  SenseTangentialVelocityMagnitude=off  NormalTransitionRegionWidth=1e-5  NormalTransitionRegionWidthUnits=m
  Obj : PMIOPort  Side=Left
  Gripper : PMIOPort  Port=2  Side=Right
  ConveyerOri : PMIOPort  Port=3  Side=Right
  ConveyerDest : PMIOPort  Port=4  Side=Right
  connections:
  BBRBall/LConn1 -- BBRConveyerDest/LConn1 -- BBRConveyerOri/LConn1 -- BBRGripper/LConn1
  ConveyerOri/RConn1 -- BBRConveyerOri/RConn1
  BBRBall/RConn1 -- BBR/RConn1
  Gripper/RConn1 -- BBRGripper/RConn1
  BBR/LConn1 -- Obj/RConn1
  BBRConveyerDest/RConn1 -- ConveyerDest/RConn1

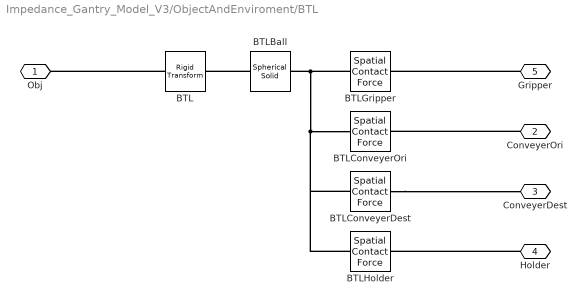
== system Impedance_Gantry_Model_V3/ObjectAndEnviroment/BTL ==
  BTL : sm_lib/Frames and Transforms/Rigid Transform  TranslationMethod=Cartesian  TranslationStandardOffset=0  TranslationLengthUnit=mm  TranslationStandardAxis=+Z  TranslationCartesianOffset=[25 25 30]  TranslationROffset=0  TranslationROffsetUnits=m  TranslationZOffset=0  TranslationZOffsetUnits=m  TranslationThetaOffset=0  TranslationThetaOffsetUnits=deg  RotationMethod=None  RotationAngleUnits=deg  RotationStandardAxis=+Z  RotationAngle=0.0  RotationArbitraryAxis=[0 0 1]  FollAlignAxisA=+X  BaseAlignAxisA=+Y  FollAlignAxisB=+Y  BaseAlignAxisB=+Z  RotationSequenceAxes=FollowerAxes  RotationSequence=XYX  RotationSequenceAngles=[0 0 0]  RotationSequenceAnglesUnits=deg  RotationMatrix=[1 0 0; 0 1 0; 0 0 1]
  BTLBall : sm_lib/Body Elements/Spherical Solid  GraphicAmbientColor=[0.15 0.15 0.15 1.0]  BasedOnType=Density  CenterOfMass=[0 0 0]  CenterOfMassUnits=m  GraphicDiffuseColor=[0.5 0.5 0.5]  Density=1000  DensityUnits=kg/m^3  DoExposeReferenceFrame=on  GraphicEmissiveColor=[0.0 0.0 0.0 1.0]  ExportEntireGeometry=on  SerializedExposedGeometries=<ExposedGeometries><ExposedGeometry><RawGeometryId>entire</RawGeometryId><ExposedGeometryId>G</ExposedGeometryId></ExposedGeometry></ExposedGeometries>  SerializedFrames=<Frames/>  MarkerShape=Sphere  MarkerSize=10  GraphicType=FromGeometry  InertiaType=CalculateFromGeometry  Mass=1  MassUnits=kg  MomentsOfInertia=[1 1 1]  MomentsOfInertiaUnits=kg*m^2  GraphicOpacity=1.0  ProductsOfInertia=[0 0 0]  ProductsOfInertiaUnits=kg*m^2  GraphicShininess=75  GraphicSpecularColor=[0.5 0.5 0.5 1.0]  SphereRadius=1  SphereRadiusUnits=mm  GraphicVisPropType=SimpleVisualProperties
  BTLConveyerDest : sm_lib/Forces and Torques/Spatial Contact Force  CoefficientOfDynamicFriction=0.5  CoefficientOfStaticFriction=0.5  SenseContactBaseRotation=off  SenseContactBaseTranslation=off  NormalDamping=30  NormalDampingUnits=N/(m/s)  SenseContactFollowerRotation=off  SenseContactFollowerTranslation=off  SenseContactSignal=off  NormalStiffness=1e4  NormalStiffnessUnits=N/m  FrictionalCriticalVelocity=1e-3  FrictionalCriticalVelocityUnits=m/s  ZeroCrossDetectContactStartAndEnd=off  FrictionType=SmoothStickSlip  SenseFrictionalForceMagnitude=off  SenseNormalForceMagnitude=off  NormalForceType=SmoothSpringDamper  SenseNormalVelocity=off  SenseSeparationDistance=off  SenseTangentialVelocity=off  SenseTangentialVelocityMagnitude=off  NormalTransitionRegionWidth=1e-5  NormalTransitionRegionWidthUnits=m
  BTLConveyerOri : sm_lib/Forces and Torques/Spatial Contact Force  CoefficientOfDynamicFriction=0.5  CoefficientOfStaticFriction=0.5  SenseContactBaseRotation=off  SenseContactBaseTranslation=off  NormalDamping=30  NormalDampingUnits=N/(m/s)  SenseContactFollowerRotation=off  SenseContactFollowerTranslation=off  SenseContactSignal=off  NormalStiffness=1e4  NormalStiffnessUnits=N/m  FrictionalCriticalVelocity=1e-3  FrictionalCriticalVelocityUnits=m/s  ZeroCrossDetectContactStartAndEnd=off  FrictionType=SmoothStickSlip  SenseFrictionalForceMagnitude=off  SenseNormalForceMagnitude=off  NormalForceType=SmoothSpringDamper  SenseNormalVelocity=off  SenseSeparationDistance=off  SenseTangentialVelocity=off  SenseTangentialVelocityMagnitude=off  NormalTransitionRegionWidth=1e-5  NormalTransitionRegionWidthUnits=m
  BTLGripper : sm_lib/Forces and Torques/Spatial Contact Force  CoefficientOfDynamicFriction=0.5  CoefficientOfStaticFriction=0.5  SenseContactBaseRotation=off  SenseContactBaseTranslation=off  NormalDamping=0  NormalDampingUnits=N/(m/s)  SenseContactFollowerRotation=off  SenseContactFollowerTranslation=off  SenseContactSignal=off  NormalStiffness=1e4  NormalStiffnessUnits=N/m  FrictionalCriticalVelocity=1e-3  FrictionalCriticalVelocityUnits=m/s  ZeroCrossDetectContactStartAndEnd=off  FrictionType=SmoothStickSlip  SenseFrictionalForceMagnitude=off  SenseNormalForceMagnitude=off  NormalForceType=SmoothSpringDamper  SenseNormalVelocity=off  SenseSeparationDistance=off  SenseTangentialVelocity=off  SenseTangentialVelocityMagnitude=off  NormalTransitionRegionWidth=1e-5  NormalTransitionRegionWidthUnits=m
  BTLHolder : sm_lib/Forces and Torques/Spatial Contact Force  CoefficientOfDynamicFriction=0.5  CoefficientOfStaticFriction=0.5  SenseContactBaseRotation=off  SenseContactBaseTranslation=off  NormalDamping=0  NormalDampingUnits=N/(m/s)  SenseContactFollowerRotation=off  SenseContactFollowerTranslation=off  SenseContactSignal=off  NormalStiffness=1e4  NormalStiffnessUnits=N/m  FrictionalCriticalVelocity=1e-3  FrictionalCriticalVelocityUnits=m/s  ZeroCrossDetectContactStartAndEnd=off  FrictionType=SmoothStickSlip  SenseFrictionalForceMagnitude=off  SenseNormalForceMagnitude=off  NormalForceType=SmoothSpringDamper  SenseNormalVelocity=off  SenseSeparationDistance=off  SenseTangentialVelocity=off  SenseTangentialVelocityMagnitude=off  NormalTransitionRegionWidth=1e-5  NormalTransitionRegionWidthUnits=m
  Obj : PMIOPort  Side=Left
  ConveyerOri : PMIOPort  Port=2  Side=Right
  ConveyerDest : PMIOPort  Port=3  Side=Right
  Holder : PMIOPort  Port=4  Side=Right
  Gripper : PMIOPort  Port=5  Side=Right
  connections:
  BTLBall/RConn1 -- BTL/RConn1
  BTLGripper/LConn1 -- BTLConveyerDest/LConn1 -- BTLHolder/LConn1 -- BTLConveyerOri/LConn1 -- BTLBall/LConn1
  BTL/LConn1 -- Obj/RConn1
  ConveyerOri/RConn1 -- BTLConveyerOri/RConn1
  Gripper/RConn1 -- BTLGripper/RConn1
  Holder/RConn1 -- BTLHolder/RConn1
  BTLConveyerDest/RConn1 -- ConveyerDest/RConn1

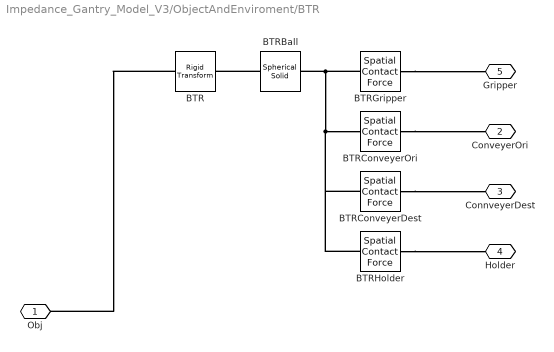
== system Impedance_Gantry_Model_V3/ObjectAndEnviroment/BTR ==
  BTR : sm_lib/Frames and Transforms/Rigid Transform  TranslationMethod=Cartesian  TranslationStandardOffset=0  TranslationLengthUnit=mm  TranslationStandardAxis=+Z  TranslationCartesianOffset=[25 0 30]  TranslationROffset=0  TranslationROffsetUnits=m  TranslationZOffset=0  TranslationZOffsetUnits=m  TranslationThetaOffset=0  TranslationThetaOffsetUnits=deg  RotationMethod=None  RotationAngleUnits=deg  RotationStandardAxis=+Z  RotationAngle=0.0  RotationArbitraryAxis=[0 0 1]  FollAlignAxisA=+X  BaseAlignAxisA=+Y  FollAlignAxisB=+Y  BaseAlignAxisB=+Z  RotationSequenceAxes=FollowerAxes  RotationSequence=XYX  RotationSequenceAngles=[0 0 0]  RotationSequenceAnglesUnits=deg  RotationMatrix=[1 0 0; 0 1 0; 0 0 1]
  BTRBall : sm_lib/Body Elements/Spherical Solid  GraphicAmbientColor=[0.15 0.15 0.15 1.0]  BasedOnType=Density  CenterOfMass=[0 0 0]  CenterOfMassUnits=m  GraphicDiffuseColor=[0.5 0.5 0.5]  Density=1000  DensityUnits=kg/m^3  DoExposeReferenceFrame=on  GraphicEmissiveColor=[0.0 0.0 0.0 1.0]  ExportEntireGeometry=on  SerializedExposedGeometries=<ExposedGeometries><ExposedGeometry><RawGeometryId>entire</RawGeometryId><ExposedGeometryId>G</ExposedGeometryId></ExposedGeometry></ExposedGeometries>  SerializedFrames=<Frames/>  MarkerShape=Sphere  MarkerSize=10  GraphicType=FromGeometry  InertiaType=CalculateFromGeometry  Mass=1  MassUnits=kg  MomentsOfInertia=[1 1 1]  MomentsOfInertiaUnits=kg*m^2  GraphicOpacity=1.0  ProductsOfInertia=[0 0 0]  ProductsOfInertiaUnits=kg*m^2  GraphicShininess=75  GraphicSpecularColor=[0.5 0.5 0.5 1.0]  SphereRadius=1  SphereRadiusUnits=mm  GraphicVisPropType=SimpleVisualProperties
  BTRConveyerDest : sm_lib/Forces and Torques/Spatial Contact Force  CoefficientOfDynamicFriction=0.5  CoefficientOfStaticFriction=0.5  SenseContactBaseRotation=off  SenseContactBaseTranslation=off  NormalDamping=30  NormalDampingUnits=N/(m/s)  SenseContactFollowerRotation=off  SenseContactFollowerTranslation=off  SenseContactSignal=off  NormalStiffness=1e4  NormalStiffnessUnits=N/m  FrictionalCriticalVelocity=1e-3  FrictionalCriticalVelocityUnits=m/s  ZeroCrossDetectContactStartAndEnd=off  FrictionType=SmoothStickSlip  SenseFrictionalForceMagnitude=off  SenseNormalForceMagnitude=off  NormalForceType=SmoothSpringDamper  SenseNormalVelocity=off  SenseSeparationDistance=off  SenseTangentialVelocity=off  SenseTangentialVelocityMagnitude=off  NormalTransitionRegionWidth=1e-5  NormalTransitionRegionWidthUnits=m
  BTRConveyerOri : sm_lib/Forces and Torques/Spatial Contact Force  CoefficientOfDynamicFriction=0.5  CoefficientOfStaticFriction=0.5  SenseContactBaseRotation=off  SenseContactBaseTranslation=off  NormalDamping=30  NormalDampingUnits=N/(m/s)  SenseContactFollowerRotation=off  SenseContactFollowerTranslation=off  SenseContactSignal=off  NormalStiffness=1e4  NormalStiffnessUnits=N/m  FrictionalCriticalVelocity=1e-3  FrictionalCriticalVelocityUnits=m/s  ZeroCrossDetectContactStartAndEnd=off  FrictionType=SmoothStickSlip  SenseFrictionalForceMagnitude=off  SenseNormalForceMagnitude=off  NormalForceType=SmoothSpringDamper  SenseNormalVelocity=off  SenseSeparationDistance=off  SenseTangentialVelocity=off  SenseTangentialVelocityMagnitude=off  NormalTransitionRegionWidth=1e-5  NormalTransitionRegionWidthUnits=m
  BTRGripper : sm_lib/Forces and Torques/Spatial Contact Force  CoefficientOfDynamicFriction=0.5  CoefficientOfStaticFriction=0.5  SenseContactBaseRotation=off  SenseContactBaseTranslation=off  NormalDamping=0  NormalDampingUnits=N/(m/s)  SenseContactFollowerRotation=off  SenseContactFollowerTranslation=off  SenseContactSignal=off  NormalStiffness=1e4  NormalStiffnessUnits=N/m  FrictionalCriticalVelocity=1e-3  FrictionalCriticalVelocityUnits=m/s  ZeroCrossDetectContactStartAndEnd=off  FrictionType=SmoothStickSlip  SenseFrictionalForceMagnitude=off  SenseNormalForceMagnitude=off  NormalForceType=SmoothSpringDamper  SenseNormalVelocity=off  SenseSeparationDistance=off  SenseTangentialVelocity=off  SenseTangentialVelocityMagnitude=off  NormalTransitionRegionWidth=1e-5  NormalTransitionRegionWidthUnits=m
  BTRHolder : sm_lib/Forces and Torques/Spatial Contact Force  CoefficientOfDynamicFriction=0.5  CoefficientOfStaticFriction=0.5  SenseContactBaseRotation=off  SenseContactBaseTranslation=off  NormalDamping=0  NormalDampingUnits=N/(m/s)  SenseContactFollowerRotation=off  SenseContactFollowerTranslation=off  SenseContactSignal=off  NormalStiffness=1e4  NormalStiffnessUnits=N/m  FrictionalCriticalVelocity=1e-3  FrictionalCriticalVelocityUnits=m/s  ZeroCrossDetectContactStartAndEnd=off  FrictionType=SmoothStickSlip  SenseFrictionalForceMagnitude=off  SenseNormalForceMagnitude=off  NormalForceType=SmoothSpringDamper  SenseNormalVelocity=off  SenseSeparationDistance=off  SenseTangentialVelocity=off  SenseTangentialVelocityMagnitude=off  NormalTransitionRegionWidth=1e-5  NormalTransitionRegionWidthUnits=m
  Obj : PMIOPort  Side=Left
  ConveyerOri : PMIOPort  Port=2  Side=Right
  ConnveyerDest : PMIOPort  Port=3  Side=Right
  Holder : PMIOPort  Port=4  Side=Right
  Gripper : PMIOPort  Port=5  Side=Right
  connections:
  BTRConveyerDest/RConn1 -- ConnveyerDest/RConn1
  BTRGripper/LConn1 -- BTRConveyerDest/LConn1 -- BTRHolder/LConn1 -- BTRConveyerOri/LConn1 -- BTRBall/LConn1
  BTRBall/RConn1 -- BTR/RConn1
  BTR/LConn1 -- Obj/RConn1
  BTRHolder/RConn1 -- Holder/RConn1
  BTRGripper/RConn1 -- Gripper/RConn1
  BTRConveyerOri/RConn1 -- ConveyerOri/RConn1

== system Impedance_Gantry_Model_V3/ObjectAndEnviroment/FBL ==
  FBL : sm_lib/Frames and Transforms/Rigid Transform  TranslationMethod=Cartesian  TranslationStandardOffset=0  TranslationLengthUnit=mm  TranslationStandardAxis=+Z  TranslationCartesianOffset=[0 25 0]  TranslationROffset=0  TranslationROffsetUnits=m  TranslationZOffset=0  TranslationZOffsetUnits=m  TranslationThetaOffset=0  TranslationThetaOffsetUnits=deg  RotationMethod=None  RotationAngleUnits=deg  RotationStandardAxis=+Z  RotationAngle=0.0  RotationArbitraryAxis=[0 0 1]  FollAlignAxisA=+X  BaseAlignAxisA=+Y  FollAlignAxisB=+Y  BaseAlignAxisB=+Z  RotationSequenceAxes=FollowerAxes  RotationSequence=XYX  RotationSequenceAngles=[0 0 0]  RotationSequenceAnglesUnits=deg  RotationMatrix=[1 0 0; 0 1 0; 0 0 1]
  FBLBall : sm_lib/Body Elements/Spherical Solid  GraphicAmbientColor=[0.15 0.15 0.15 1.0]  BasedOnType=Density  CenterOfMass=[0 0 0]  CenterOfMassUnits=m  GraphicDiffuseColor=[0.5 0.5 0.5]  Density=1000  DensityUnits=kg/m^3  DoExposeReferenceFrame=on  GraphicEmissiveColor=[0.0 0.0 0.0 1.0]  ExportEntireGeometry=on  SerializedExposedGeometries=<ExposedGeometries><ExposedGeometry><RawGeometryId>entire</RawGeometryId><ExposedGeometryId>G</ExposedGeometryId></ExposedGeometry></ExposedGeometries>  SerializedFrames=<Frames/>  MarkerShape=Sphere  MarkerSize=10  GraphicType=FromGeometry  InertiaType=CalculateFromGeometry  Mass=1  MassUnits=kg  MomentsOfInertia=[1 1 1]  MomentsOfInertiaUnits=kg*m^2  GraphicOpacity=1.0  ProductsOfInertia=[0 0 0]  ProductsOfInertiaUnits=kg*m^2  GraphicShininess=75  GraphicSpecularColor=[0.5 0.5 0.5 1.0]  SphereRadius=1  SphereRadiusUnits=mm  GraphicVisPropType=SimpleVisualProperties
  FBLConveyerDest : sm_lib/Forces and Torques/Spatial Contact Force  CoefficientOfDynamicFriction=0.5  CoefficientOfStaticFriction=0.5  SenseContactBaseRotation=off  SenseContactBaseTranslation=off  NormalDamping=30  NormalDampingUnits=N/(m/s)  SenseContactFollowerRotation=off  SenseContactFollowerTranslation=off  SenseContactSignal=off  NormalStiffness=1e4  NormalStiffnessUnits=N/m  FrictionalCriticalVelocity=1e-3  FrictionalCriticalVelocityUnits=m/s  ZeroCrossDetectContactStartAndEnd=off  FrictionType=SmoothStickSlip  SenseFrictionalForceMagnitude=off  SenseNormalForceMagnitude=off  NormalForceType=SmoothSpringDamper  SenseNormalVelocity=off  SenseSeparationDistance=off  SenseTangentialVelocity=off  SenseTangentialVelocityMagnitude=off  NormalTransitionRegionWidth=1e-5  NormalTransitionRegionWidthUnits=m
  FBLConveyerOri : sm_lib/Forces and Torques/Spatial Contact Force  CoefficientOfDynamicFriction=0.5  CoefficientOfStaticFriction=0.5  SenseContactBaseRotation=off  SenseContactBaseTranslation=off  NormalDamping=30  NormalDampingUnits=N/(m/s)  SenseContactFollowerRotation=off  SenseContactFollowerTranslation=off  SenseContactSignal=off  NormalStiffness=1e4  NormalStiffnessUnits=N/m  FrictionalCriticalVelocity=1e-3  FrictionalCriticalVelocityUnits=m/s  ZeroCrossDetectContactStartAndEnd=off  FrictionType=SmoothStickSlip  SenseFrictionalForceMagnitude=off  SenseNormalForceMagnitude=off  NormalForceType=SmoothSpringDamper  SenseNormalVelocity=off  SenseSeparationDistance=off  SenseTangentialVelocity=off  SenseTangentialVelocityMagnitude=off  NormalTransitionRegionWidth=1e-5  NormalTransitionRegionWidthUnits=m
  FBLGripper : sm_lib/Forces and Torques/Spatial Contact Force  CoefficientOfDynamicFriction=0.5  CoefficientOfStaticFriction=0.5  SenseContactBaseRotation=off  SenseContactBaseTranslation=off  NormalDamping=0  NormalDampingUnits=N/(m/s)  SenseContactFollowerRotation=off  SenseContactFollowerTranslation=off  SenseContactSignal=off  NormalStiffness=1e4  NormalStiffnessUnits=N/m  FrictionalCriticalVelocity=1e-3  FrictionalCriticalVelocityUnits=m/s  ZeroCrossDetectContactStartAndEnd=off  FrictionType=SmoothStickSlip  SenseFrictionalForceMagnitude=off  SenseNormalForceMagnitude=off  NormalForceType=SmoothSpringDamper  SenseNormalVelocity=off  SenseSeparationDistance=off  SenseTangentialVelocity=off  SenseTangentialVelocityMagnitude=off  NormalTransitionRegionWidth=1e-5  NormalTransitionRegionWidthUnits=m
  Gripper : PMIOPort  Side=Right
  Obj : PMIOPort  Port=2  Side=Left
  ConveyerOri : PMIOPort  Port=3  Side=Right
  ConveyerDest : PMIOPort  Port=4  Side=Right
  connections:
  FBLBall/LConn1 -- FBLConveyerDest/LConn1 -- FBLConveyerOri/LConn1 -- FBLGripper/LConn1
  FBLConveyerOri/RConn1 -- ConveyerOri/RConn1
  FBLBall/RConn1 -- FBL/RConn1
  FBL/LConn1 -- Obj/RConn1
  FBLGripper/RConn1 -- Gripper/RConn1
  FBLConveyerDest/RConn1 -- ConveyerDest/RConn1
